simulink model "controller"  (R2019b)
settings: Solver=FixedStepAuto  StartTime=0.0  StopTime=t_end  FixedStep=0.01  MaxStep=.1  RelTol=1e-3
values from neighbouring files (symbols this model uses):
  K = zeros(1,2)    [a_init_model.m]    (also in duffing_init.m)
  Ts = 30*dt    (= 0.3)    [duffing_init.m]    (also in duffing_linear.m = 10*dt; f_init_hybrid.m = 0.2)
settings Model: Creator=enrique.babio  LastModifiedBy=enrique.babio
settings DataIOCC: SaveOutput=off  SaveState=on  SaveTime=off

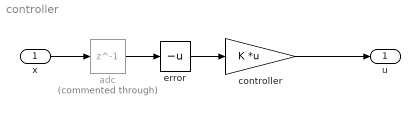
== system controller ==
  x : Inport  OutDataTypeStr=double  PortDimensions=2  SampleTime=0
  adc : Delay  Commented=through  DelayLength=1  SampleTime=Ts  StateName=adcDelay
  controller : Gain  Gain=K  Multiplication=Matrix(K*u)
  error : UnaryMinus
  u : Outport  OutDataTypeStr=double  PortDimensions=1
  wires:
  error/1 -> controller/1
  controller/1 -> u/1
  x/1 -> adc/1
  adc/1 -> error/1
